simulink model "Displays_ARES_Sim"  (R2019b)
settings: Solver=FixedStepAuto  StartTime=0  StopTime=500  RelTol=1e-3  EnableMultiTasking=on
values from neighbouring files (symbols this model uses):
  Avail_Mode = 2    [Init_Vars_ARES_Sim.m]    (also in Init_Vars_ARES_Sim_SR.m = 0; Init_Vars_ARES_Sim_SR_Michael.m = 0)
  quad_s = 1    [Init_Vars_ARES_Sim.m]    (also in Init_Vars_ARES_Sim_SR.m; Init_Vars_ARES_Sim_SR_Michael.m)
  xLP0 = x0    (= 12000)    [Init_Vars_ARES_Sim.m]    (also in Init_Vars_ARES_Sim_SR.m; Init_Vars_ARES_Sim_SR_Michael.m)
  yLP0 = y0 + 1350    (= 13350)    [Init_Vars_ARES_Sim.m]    (also in Init_Vars_ARES_Sim_SR.m = 10950; Init_Vars_ARES_Sim_SR_Michael.m = 10950)
undefined symbols (not defined in the file or in its folder): LPs, var
libraries: vrlib x37, simulink x5, visionsources x3, simulink_extras x1, aerolibanimutils x1
(part 2 of 2)

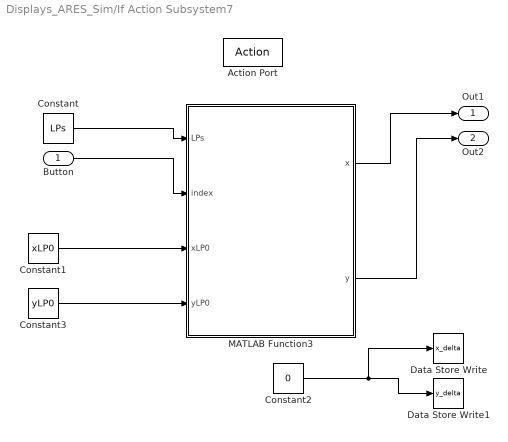
== system Displays_ARES_Sim/If Action Subsystem7 ==
  Button : Inport
  Action Port : ActionPort  ActionPortLabel=if(u1 ~= 0)
  Constant : Constant  Value=LPs
  Constant1 : Constant  Value=xLP0
  Constant2 : Constant  Value=0
  Constant3 : Constant  Value=yLP0
  Data Store Write : DataStoreWrite  DataStoreName=x_delta
  Data Store Write1 : DataStoreWrite  DataStoreName=y_delta
  MATLAB Function3 : MATLAB Function  TreatAsAtomicUnit=on
  Out1 : Outport  InitialOutput=[xLP0]  VectorParamsAs1DForOutWhenUnconnected=off
  Out2 : Outport  Port=2  InitialOutput=[yLP0]  VectorParamsAs1DForOutWhenUnconnected=off
  wires:
  Constant1/1 -> MATLAB Function3/3(xLP0)
  Constant/1 -> MATLAB Function3/1(LPs)
  Constant3/1 -> MATLAB Function3/4(yLP0)
  Button/1 -> MATLAB Function3/2(index)
  MATLAB Function3/1(x) -> Out1/1
  MATLAB Function3/2(y) -> Out2/1
  Constant2/1 -> Data Store Write1/1, Data Store Write/1

== system Displays_ARES_Sim/If Action Subsystem8 ==
  Action Port : ActionPort  ActionPortLabel=if(u1 < 0.0003)

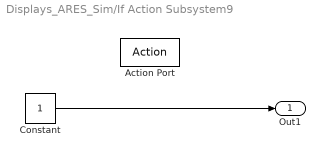
== system Displays_ARES_Sim/If Action Subsystem9 ==
  Action Port : ActionPort  ActionPortLabel=if(u1 ==1 & u2 ==1)
  Constant : Constant
  Out1 : Outport  InitialOutput=[0]  VectorParamsAs1DForOutWhenUnconnected=off
  wires:
  Constant/1 -> Out1/1

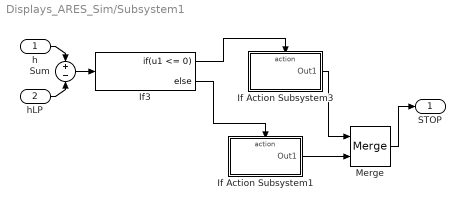
== system Displays_ARES_Sim/Subsystem1 ==
  h : Inport
  hLP : Inport  Port=2
  If Action Subsystem1 : Subsystem  TreatAsAtomicUnit=on
  If Action Subsystem3 : Subsystem  TreatAsAtomicUnit=on
  If3 : If  IfExpression=u1 <= 0  ZeroCross=off
  Merge : Merge
  Sum : Sum  Inputs=+-
  STOP : Outport  VectorParamsAs1DForOutWhenUnconnected=off
  wires:
  If3/1 -> If Action Subsystem3/Action
  Sum/1 -> If3/1
  h/1 -> Sum/1
  hLP/1 -> Sum/2
  If3/2 -> If Action Subsystem1/Action
  If Action Subsystem3/1(Out1) -> Merge/1
  Merge/1 -> STOP/1
  If Action Subsystem1/1(Out1) -> Merge/2

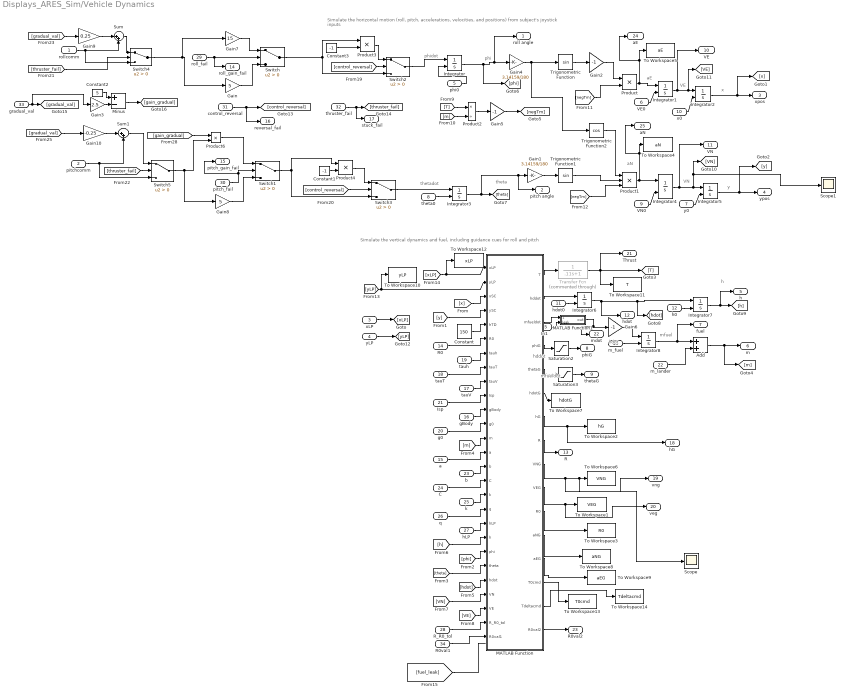
== system Displays_ARES_Sim/Vehicle Dynamics  ==
  note: Simulate the horizontal motion (roll, pitch, accelerations, velocities, and positions) from subject's joystick inputs
  note: Simulate the vertical dynamics and fuel, including guidance cues for roll and pitch
  note: mfuel
  note: mfueldot
  note: h
  note: hdot
  note: hddot
  note: aN
  note: x
  note: VE
  note: aE
  note: phi
  note: phidot
  note: theta
  note: thetadot
  note: y
  note: VN
  rollcomm : Inport
  "pitchcomm " : Inport  Port=2
  xLP : Inport  Port=3
  yLP : Inport  Port=4
  phi0 : Inport  Port=5
  VE0 : Inport  Port=6
  y0 : Inport  Port=7
  "theta0 " : Inport  Port=8
  VN0 : Inport  Port=9
  "x0 " : Inport  Port=10
  hdot0 : Inport  Port=11
  h0 : Inport  Port=12
  m_fuel : Inport  Port=13
  R0 : Inport  Port=14
  a : Inport  Port=15
  gBody : Inport  Port=16
  tauV : Inport  Port=17
  tauT : Inport  Port=18
  tauh : Inport  Port=19
  g0 : Inport  Port=20
  Isp : Inport  Port=21
  m_lander : Inport  Port=22
  "b " : Inport  Port=23
  C : Inport  Port=24
  k : Inport  Port=25
  q : Inport  Port=26
  hLP : Inport  Port=27
  R_R0_tol : Inport  Port=28
  roll_fail : Inport  Port=29
  pitch_fail : Inport  Port=30
  control_reversal : Inport  Port=31
  thruster_fail : Inport  Port=32
  gradual_val : Inport  Port=33
  R0val1 : Inport  Port=34
  In1 : Inport  Port=35
  Add : Sum
  Constant : Constant  Value=150
  Constant1 : Constant  Value=-1
  Constant2 : Constant  Value=5
  Constant3 : Constant  Value=-1
  Gain : Gain  Gain=5
  Gain1 : Gain  Gain=3.14159/180
  Gain10 : Gain  Gain=-0.25
  Gain2 : Gain  Gain=-1
  Gain3 : Gain  Gain=2.5
  Gain4 : Gain  Gain=3.14159/180
  Gain5 : Gain  Gain=-1
  Gain6 : Gain  Gain=-1
  Gain7 : Gain  Gain=15
  Gain8 : Gain  Gain=5
  Gain9 : Gain  Gain=0.25
  Integrator{,1,6..8} (5 alike) : Integrator  InitialConditionSource=external
  Integrator2 : Integrator  InitialConditionSource=external  InitialCondition=1000
  Integrator3 : Integrator  InitialConditionSource=external  InitialCondition=-16
  Integrator4 : Integrator  InitialConditionSource=external  InitialCondition=var]
  Integrator5 : Integrator  InitialConditionSource=external  InitialCondition=1000
  MATLAB Function : MATLAB Function  TreatAsAtomicUnit=on  SystemSampleTime=0.1
  MATLAB Function1 : MATLAB Function  TreatAsAtomicUnit=on
  Minus : Sum  Inputs=+-
  Product{,3..4,6} (4 alike) : Product
  Product1 : Product  Inputs=3
  Product2 : Product  Inputs=*/
  Saturation2 : Saturate  UpperLimit=45  LowerLimit=-45
  Saturation3 : Saturate  UpperLimit=45  LowerLimit=-45
  Scope : Scope
  Scope1 : Scope
  Sum : Sum  Inputs=|++
  Sum1 : Sum  Inputs=|++
  Switch{,1..5} (6 alike) : Switch  Criteria=u2 > Threshold
  To Workspace1 : ToWorkspace  VariableName=VEG  SaveFormat=Timeseries  SampleTime=-1
  To Workspace10 : ToWorkspace  VariableName=yLP  SaveFormat=Timeseries  SampleTime=-1
  To Workspace11 : ToWorkspace  VariableName=T  SaveFormat=Timeseries  SampleTime=-1
  To Workspace12 : ToWorkspace  VariableName=xLP  SaveFormat=Timeseries  SampleTime=-1
  To Workspace13 : ToWorkspace  VariableName=T0cmd  SaveFormat=Timeseries  SampleTime=-1
  To Workspace14 : ToWorkspace  VariableName=Tdeltacmd  SaveFormat=Timeseries  SampleTime=-1
  To Workspace2 : ToWorkspace  VariableName=hG  SaveFormat=Timeseries  SampleTime=-1
  To Workspace3 : ToWorkspace  VariableName=R0  SaveFormat=Timeseries  SampleTime=-1
  To Workspace4 : ToWorkspace  VariableName=aN  SaveFormat=Timeseries  SampleTime=-1
  To Workspace5 : ToWorkspace  VariableName=aE  SaveFormat=Timeseries  SampleTime=-1
  To Workspace6 : ToWorkspace  VariableName=VNG  SaveFormat=Timeseries  SampleTime=-1
  To Workspace7 : ToWorkspace  VariableName=hdotG  SaveFormat=Timeseries  SampleTime=-1
  To Workspace8 : ToWorkspace  VariableName=aNG  SaveFormat=Timeseries  SampleTime=-1
  To Workspace9 : ToWorkspace  VariableName=aEG  SaveFormat=Timeseries  SampleTime=-1
  Transfer Fcn : TransferFcn  Commented=through  Denominator=[.11 1]
  Trigonometric Function : Trigonometry
  Trigonometric Function1 : Trigonometry
  Trigonometric Function2 : Trigonometry  Operator=cos
  roll angle : Outport  VectorParamsAs1DForOutWhenUnconnected=off
  pitch angle : Outport  Port=2  VectorParamsAs1DForOutWhenUnconnected=off
  xpos : Outport  Port=3  VectorParamsAs1DForOutWhenUnconnected=off
  "ypos " : Outport  Port=4  VectorParamsAs1DForOutWhenUnconnected=off
  h : Outport  Port=5  VectorParamsAs1DForOutWhenUnconnected=off
  m : Outport  Port=6  VectorParamsAs1DForOutWhenUnconnected=off
  fuel : Outport  Port=7  VectorParamsAs1DForOutWhenUnconnected=off
  phiG : Outport  Port=8  VectorParamsAs1DForOutWhenUnconnected=off
  thetaG : Outport  Port=9  VectorParamsAs1DForOutWhenUnconnected=off
  VE : Outport  Port=10  VectorParamsAs1DForOutWhenUnconnected=off
  VN : Outport  Port=11  VectorParamsAs1DForOutWhenUnconnected=off
  "hdot " : Outport  Port=12  VectorParamsAs1DForOutWhenUnconnected=off
  R : Outport  Port=13  VectorParamsAs1DForOutWhenUnconnected=off
  roll_gain_fail : Outport  Port=14  VectorParamsAs1DForOutWhenUnconnected=off
  pitch_gain_fail : Outport  Port=15  VectorParamsAs1DForOutWhenUnconnected=off
  reversal_fail : Outport  Port=16  VectorParamsAs1DForOutWhenUnconnected=off
  stuck_fail : Outport  Port=17  VectorParamsAs1DForOutWhenUnconnected=off
  hG : Outport  Port=18  VectorParamsAs1DForOutWhenUnconnected=off
  "vng " : Outport  Port=19  VectorParamsAs1DForOutWhenUnconnected=off
  veg : Outport  Port=20  VectorParamsAs1DForOutWhenUnconnected=off
  Thrust : Outport  Port=21  VectorParamsAs1DForOutWhenUnconnected=off
  mdot : Outport  Port=22  VectorParamsAs1DForOutWhenUnconnected=off
  R0val2 : Outport  Port=23  VectorParamsAs1DForOutWhenUnconnected=off
  aE : Outport  Port=24  VectorParamsAs1DForOutWhenUnconnected=off
  aN : Outport  Port=25  VectorParamsAs1DForOutWhenUnconnected=off
  wires:
  Trigonometric Function/1 -> Gain2/1
  Product/1 -> aE/1, To Workspace5/1, Integrator1/1
  Integrator1/1 -> VE/1, [VE], Integrator2/1
  Integrator2/1 -> xpos/1, [x]
  Gain2/1 -> Product/1
  [negTm] -> Product1/3
  Trigonometric Function1/1 -> Product1/2
  Trigonometric Function2/1 -> Product1/1
  Integrator4/1 -> VN/1, Scope1/1, [VN], Integrator5/1
  Integrator5/1 -> "ypos "/1, [y]
  Product1/1 -> aN/1, To Workspace4/1, Integrator4/1
  MATLAB Function/2(hddot) -> Integrator6/1
  xLP/1 -> [xLP]
  yLP/1 -> [yLP]
  [x] -> MATLAB Function/3(xSC)
  [y] -> MATLAB Function/4(ySC)
  R0/1 -> MATLAB Function/6("R0 ")
  tauh/1 -> MATLAB Function/7(tauh)
  Integrator7/1 -> h/1, [h]
  Add/1 -> m/1, [m]
  Gain6/1 -> Integrator8/1
  Integrator8/1 -> fuel/1, Add/1
  m_lander/1 -> Add/2
  [T] -> Product2/1
  Product2/1 -> Gain5/1
  Gain5/1 -> [negTm]
  [negTm] -> Product/2
  phi0/1 -> Integrator/2
  VE0/1 -> Integrator1/2
  y0/1 -> Integrator5/2
  "theta0 "/1 -> Integrator3/2
  VN0/1 -> Integrator4/2
  "x0 "/1 -> Integrator2/2
  h0/1 -> Integrator7/2
  hdot0/1 -> Integrator6/2
  m_fuel/1 -> Integrator8/2
  tauT/1 -> MATLAB Function/8(tauT)
  Isp/1 -> MATLAB Function/10(Isp)
  gBody/1 -> MATLAB Function/11(gBody)
  g0/1 -> MATLAB Function/12(g0)
  [m] -> MATLAB Function/13(m)
  [h] -> MATLAB Function/20(h)
  [phi] -> MATLAB Function/21(phi)
  [hdot] -> MATLAB Function/23(hdot)
  [theta] -> MATLAB Function/22(theta)
  [VN] -> MATLAB Function/24(VN)
  [VE] -> MATLAB Function/25(VE)
  tauV/1 -> MATLAB Function/9(tauV)
  [m] -> Product2/2
  MATLAB Function/8(R) -> R/1
  Gain1/1 -> Trigonometric Function1/1
  Gain4/1 -> Trigonometric Function2/1, Trigonometric Function/1
  "b "/1 -> MATLAB Function/15(b)
  C/1 -> MATLAB Function/16(C)
  k/1 -> MATLAB Function/17(k)
  Integrator/1 -> [phi], roll angle/1, Gain4/1
  Integrator3/1 -> pitch angle/1, Gain1/1, [theta]
  Constant/1 -> MATLAB Function/5(hTD)
  hLP/1 -> MATLAB Function/19(hLP)
  q/1 -> MATLAB Function/18(q)
  a/1 -> MATLAB Function/14(a)
  MATLAB Function/4(phiG) -> Saturation2/1
  Saturation2/1 -> phiG/1
  MATLAB Function/5(thetaG) -> Saturation3/1
  Saturation3/1 -> thetaG/1
  MATLAB Function/9(VNG) -> Scope/1, "vng "/1, To Workspace6/1
  MATLAB Function/6(hdotG) -> To Workspace7/1
  MATLAB Function/7(hG) -> hG/1, To Workspace2/1
  [xLP] -> MATLAB Function/1(xLP), To Workspace12/1
  [yLP] -> To Workspace10/1, MATLAB Function/2(yLP)
  R_R0_tol/1 -> MATLAB Function/26(R_R0_tol)
  MATLAB Function/11(R0) -> To Workspace3/1
  MATLAB Function/12(aNG) -> To Workspace8/1
  MATLAB Function/13(aEG) -> To Workspace9/1
  MATLAB Function/14(T0cmd) -> To Workspace13/1
  MATLAB Function/15(Tdeltacmd) -> To Workspace14/1
  MATLAB Function/1(T) -> Transfer Fcn/1
  Integrator6/1 -> [hdot], Integrator7/1, "hdot "/1
  Gain/1 -> Switch/3
  Gain8/1 -> Switch1/3
  roll_fail/1 -> roll_gain_fail/1, Switch/2
  pitch_fail/1 -> pitch_gain_fail/1, Switch1/2
  Constant3/1 -> Product3/2
  Switch2/1 -> Integrator/1
  control_reversal/1 -> reversal_fail/1, [control_reversal]
  [control_reversal] -> Switch2/2
  Product3/1 -> Switch2/1
  Switch/1 -> Switch2/3, Product3/1
  Constant1/1 -> Product4/2
  [control_reversal] -> Switch3/2
  Product4/1 -> Switch3/1
  Switch3/1 -> Integrator3/1
  Switch1/1 -> Switch3/3, Product4/1
  Sum/1 -> Switch4/1
  thruster_fail/1 -> [thruster_fail], stuck_fail/1
  rollcomm/1 -> Sum/2, Switch4/3
  [thruster_fail] -> Switch4/2
  [thruster_fail] -> Switch5/2
  "pitchcomm "/1 -> Switch5/3, Sum1/2
  Sum1/1 -> Switch5/1
  Switch4/1 -> Gain7/1, Gain/1
  Gain9/1 -> Sum/1
  [gradual_val] -> Gain9/1
  [gradual_val] -> Gain10/1
  Gain10/1 -> Sum1/1
  Product6/1 -> Switch1/1
  Switch5/1 -> Product6/2, Gain8/1
  gradual_val/1 -> Gain3/1, [gradual_val]
  Constant2/1 -> Minus/1
  Gain3/1 -> Minus/2
  Minus/1 -> [gain_gradual]
  [gain_gradual] -> Product6/1
  MATLAB Function/10(VEG) -> veg/1, To Workspace1/1
  Transfer Fcn/1 -> To Workspace11/1, Thrust/1, [T]
  Gain7/1 -> Switch/1
  R0val1/1 -> MATLAB Function/27(R0val1)
  MATLAB Function/16(R0val2) -> R0val2/1
  [fuel_leak] -> ?
  MATLAB Function/3(mfueldot) -> MATLAB Function1/1(mfueldot)
  MATLAB Function1/1(out) -> mdot/1, Gain6/1
  In1/1 -> MATLAB Function1/2(leak)

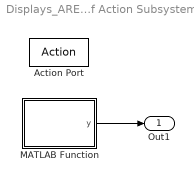
== system Displays_ARES_Sim/If Action Subsystem5/If Action Subsystem1 ==
  Action Port : ActionPort  ActionPortLabel=elseif(u1 == 2)
  MATLAB Function : MATLAB Function  TreatAsAtomicUnit=on
  Out1 : Outport  VectorParamsAs1DForOutWhenUnconnected=off
  wires:
  MATLAB Function/1(y) -> Out1/1

== system Displays_ARES_Sim/If Action Subsystem5/If Action Subsystem2 ==
  Action Port : ActionPort  ActionPortLabel=if(u1 == 1)
  MATLAB Function : MATLAB Function  TreatAsAtomicUnit=on
  Out1 : Outport  VectorParamsAs1DForOutWhenUnconnected=off
  wires:
  MATLAB Function/1(y) -> Out1/1

== system Displays_ARES_Sim/If Action Subsystem5/If Action Subsystem3 ==
  Action Port : ActionPort  ActionPortLabel=elseif( u1 == 3)
  MATLAB Function : MATLAB Function  TreatAsAtomicUnit=on
  Out1 : Outport  VectorParamsAs1DForOutWhenUnconnected=off
  wires:
  MATLAB Function/1(y) -> Out1/1

== system Displays_ARES_Sim/If Action Subsystem5/If Action Subsystem4 ==
  Action Port : ActionPort  ActionPortLabel=elseif( u1 == 4)
  MATLAB Function : MATLAB Function  TreatAsAtomicUnit=on
  Out1 : Outport  VectorParamsAs1DForOutWhenUnconnected=off
  wires:
  MATLAB Function/1(y) -> Out1/1

== system Displays_ARES_Sim/If Action Subsystem5/If Action Subsystem5 ==
  Action Port : ActionPort  ActionPortLabel=elseif(u1==5)
  MATLAB Function : MATLAB Function  TreatAsAtomicUnit=on
  Out1 : Outport  VectorParamsAs1DForOutWhenUnconnected=off
  wires:
  MATLAB Function/1(y) -> Out1/1

== system Displays_ARES_Sim/If Action Subsystem5/If Action Subsystem6 ==
  Action Port : ActionPort  ActionPortLabel=elseif(u1==6)
  MATLAB Function : MATLAB Function  TreatAsAtomicUnit=on
  Out1 : Outport  VectorParamsAs1DForOutWhenUnconnected=off
  wires:
  MATLAB Function/1(y) -> Out1/1

== system Displays_ARES_Sim/Subsystem1/If Action Subsystem1 ==
  Action Port : ActionPort  ActionPortLabel=else
  Constant1 : Constant  Value=0
  Out1 : Outport  VectorParamsAs1DForOutWhenUnconnected=off
  wires:
  Constant1/1 -> Out1/1

== system Displays_ARES_Sim/Subsystem1/If Action Subsystem3 ==
  Action Port : ActionPort  ActionPortLabel=if(u1 <= 0)
  Constant1 : Constant
  Out1 : Outport  InitialOutput=[0]  VectorParamsAs1DForOutWhenUnconnected=off
  wires:
  Constant1/1 -> Out1/1

== matlab function Displays_ARES_Sim/If Action Subsystem/Fuel Gauge ==
  data: fuel input; pts output; m_fuel0 input; fuel_percent output
function [pts,fuel_percent] = fcn( fuel, m_fuel0 )
pts = [0 0 0];
fuelH = fuel/m_fuel0;
fuel_percent = fuelH;
p9 = [ 1 fuelH 1];

pts = [p9];

== matlab function Displays_ARES_Sim/Vehicle Dynamics /MATLAB Function ==
  settings: updateMethod=DISCRETE
  data: xLP input; T output; yLP input; xSC input; ySC input; hTD input; R0 input; tauh input; tauT input; tauV input; Isp input; gBody input; g0 input; m input; a input; b input; C input; k input; q input; hLP input; hddot output; mfueldot output; h input; phi input; theta input; hdot input; VN input; VE input; phiG output; thetaG output; hdotG output; hG output; R output; VNG output; VEG output; R_R0_tol input; R0 output; aNG output; aEG output; T0cmd output; Tdeltacmd output; R0val data_store_memory; R0val1 input; R0val2 output
function [T, hddot, mfueldot, phiG, thetaG, hdotG, hG, R, VNG, VEG,R0,aNG,aEG,T0cmd,Tdeltacmd,R0val2]= fcn(xLP, yLP, xSC, ySC, hTD, R0,tauh, tauT, tauV, Isp, gBody, g0, m, a, b, C, k, q, hLP, h, phi, theta, hdot, VN, VE, R_R0_tol,R0val1)


%% Guidance 
ySC_LP = ySC - yLP; % north distance in s/c to LP
xSC_LP = xSC - xLP; % east distance in s/c to LP
hRel = h - hLP;
psi = 0;

R = sqrt(xSC_LP^2 + ySC_LP^2);

R0 = R0val1;

% Our added logic to deal with cases where you are farther away from LP
% than when you started the landing
if (R/R0val1) > (exp(1)^2 - R_R0_tol)
    % Change R0 to your actual range because VN blows up  if R/R0 is
    % greater than e^2. This will create a "new" simulation (new initial
    % range that you are evaluating from). Essentially  restarting the
    % simulation where the previous state left of
    % Set R0 global to the current range value (redefine R0) (new R0 for
    % the remaining time steps)
    R0val2 = R;
    % Changes R0 for the current time step
    R0 = R;
%     Rchecker = 1;
else
    R0val2 = R0val1;
end

% changed from -xSC and -ySC
angleLP = 180/pi*atan2(-xSC_LP,-ySC_LP);
Rdot = -VN*cosd(angleLP) - VE*sind(angleLP);

% Hdot Guidance
if hRel >= 150
    hG = C + (((hTD-C)^log(sqrt(R/R0)))/k)^(1/(log(sqrt(R/R0))-1));     % ft, Equation 10
    if hG > 1000
        hG = 1000;
    end
    hdotG = (a*hG + b) + (hG - hRel)/tauh;                               % ft/s, Equation 11
else
    hG = hRel;     % ft, not a real thing, just a place holder for once we get below 150 ft since hG is no longer defined
    hdotG = -3;                                                       % ft, if below 150 ft, just descend at -3 ft/s
end

% Add in a limit that if we are too far away (>Rlim) but too low (<150ft),
% go into hover (this is our own personal addition, not from Bilimoria)
Rlim = 100; %50     % ft, the limit for how small the range has to be for us to continue to descend if we are below 150 ft
if hRel < hTD && R > Rlim
    hdotG = 0;  % go into a hover (i.e. hdotG=0)
end

% Limit hdotG to between 0 and -30 f/s
if hdotG > 0
    hdotG = 0;
elseif hdotG < -16
    hdotG = -16;
end

% Define a deadband that will be added in on the Tdetlacmd when assum
hdot_deadband = 0.1;                % ft/s
% The commanded vertical velocity will always be the guidance vertical velocity

hdotcmd = hdotG;        % assuming this to be the case, need to verify

%% hdotG failure...
% if no_fail 
% hdotcmd = hdotG;        % assuming this to be the case, need to verify
% else
%     hdotcmd = 1.3*hdot
% end
%% 

% thrust command
T0cmd = m*gBody/(cosd(theta)*cosd(phi));       % ft-lbs (like N), Equation 1, primary thrust command to counteract weight of the vehicle
% change in thrust command
Tdeltacmd = m/(cosd(theta)*cosd(phi)) * (hdotcmd-hdot)/tauT;    % ft-lbs (like N), Equation 2, secondary thrust command to adjust descent rate
% Add a deadband in on the Tdetlacmd
if abs(hdotcmd-hdot) < hdot_deadband
    Tdeltacmd = 0;
end
T = T0cmd + Tdeltacmd; % ft-lbs (like N), total thrust command
% Constrain thrust between 10% and 60% of max operational thrust (10,000 lbf)
if T > 6000
    T = 6000;
end
if T < 1000
    T = 1000;
end
hddot = T/m * cosd(phi)*cosd(theta) - gBody;    % ft/s^2, vertical acceleration
% Change in vehicle mass
mfueldot = T/(Isp*g0);      % slugs/s, fuel consumption rate, assumes ideal rocket equation
% mdot = -mfueldot;           % slug/s
% if fuel_leak==1
%     mfueldot=1.5*mfueldot;
% end 

% Velocity guidance (North and East)
VNG = ySC_LP*q*(1-log(sqrt(R/R0)));     % ft/s, Equation 13a
VEG = xSC_LP*q*(1-log(sqrt(R/R0)));     % ft/s, Equation 13b

% acceleration Guidance (North and East)
% Set x acceleration equal to zero if x = 0
if ySC_LP == 0
    aNG = 0;
else
    aNG = (VN*VNG/ySC_LP + q*(-1)*ySC_LP*Rdot/(2*R)) + (VNG - VN)/tauV;  % ft/s^2, Equation 15a
end
% Set y acceleration equal to zero if y = 0
if xSC_LP == 0
    aEG = 0;
else
    aEG = (VE*VEG/xSC_LP + q*(-1)*xSC_LP*Rdot/(2*R)) + (VEG - VE)/tauV;  % ft/s^2, Equation 15b
end

temp = -m/T * (aNG*sind(psi) - aEG*cosd(psi));
if temp > 1
    temp = 1;
elseif temp < -1
    temp = -1;
end

% % roll Guidance
phiG = asind(temp);   % deg, (positive is nose up), Equation 17a
% % Limit phiG by +/- 45 deg
if phiG > 45
    phiG = 45;
elseif phiG < -45
    phiG = -45;
end

% Limit phiG by +/- 30 deg to try and make trials longer
% if phiG > 30
%     phiG = 30;
% elseif phiG < -30
%     phiG = -30;
% end


temp2 = -m/(T*cosd(phiG)) * (aNG*cosd(psi) + aEG*sind(psi));
if temp2 > 1
    temp2 = 1;
elseif temp2 < -1
    temp2 = -1;
end

% pitch Guidance
thetaG = asind(temp2);   % deg, (positive is nose up), Equation 17b
% % Limit thetaG by +/- 45 deg
if thetaG > 45
    thetaG = 45;
elseif thetaG < -45
    thetaG = -45;

% Limit thetaG by +/- 30 deg
% if thetaG > 30
%     thetaG = 30;
% elseif thetaG < -30
%     thetaG = -30;
    
end

== matlab function Displays_ARES_Sim/Background Translation ==
  data: pitch input; pts output; roll input
%%%%%%%%%%%%%%%%%%%%%%%%%%%%%%%%%%%%%
% This function is used to define the translation of the guidance cues
% Elliott Davis 
% Edited: 4/30/18
% Joshua Seedorf
% Edited: 1/21/20
% Modified transformation to display roll correctly
%%%%%%%%%%%%%%%%%%%%%%%%%%%%%%%%%%%%%
function pts   = fcn( pitch, roll )

% Roll and Pitch
% x = xy(1);
% y = xy(2);

%% Roll Correction
% X-component
x = (0.1045)*pitch*sind(roll);
% Y-component
y = (0.1045)*pitch*cosd(roll);

% Output for VR sink (y,z)
% pts = [0 (-pitch-25) -.5];
pts = [x -y-25 -0.5];

== matlab function Displays_ARES_Sim/Rotations ==
  data: xy input; pts output
%%%%%%%%%%%%%%%%%%%%%%%%%%%%%%%%%%%%%
% This function is used to define the rotation of pitch bars
% Elliott Davis 
% Edited: 4/30/18
%%%%%%%%%%%%%%%%%%%%%%%%%%%%%%%%%%%%%
function pts   = fcn( xy )

% Roll and Pitch
x = xy(1);
y = xy(2);

% Output for VR sink (z,angle)
pts = [ 1 x/5.75];

== matlab function Displays_ARES_Sim/Guidance Cross ==
  data: thetaG input; pts output; phiG input; theta input; phi input
%%%%%%%%%%%%%%%%%%%%%%%%%%%%%%%%%%%%%
% This function is used to define the translation of the guidance cues
% Elliott Davis 
% Edited: 4/30/18
%%%%%%%%%%%%%%%%%%%%%%%%%%%%%%%%%%%%%
function pts = fcn( thetaG, phiG, theta, phi )

% Input pitch/roll and respective guidance
x = phiG;
y = thetaG;
out1 = x-phi;
out2 = y-theta;

% Define limits on the outputs
if out1 >= 4.5
    out1 = 4.5;
elseif out1 <= -4.5 
    out1 = -4.5;
end 

if out2 >= 4.5
    out2 = 4.5;
elseif out2 <= -4.5 
    out2 = -4.5;
end 

% Output for VR sink (x,y,z)
pts = [out1 out2 .001];

== matlab function Displays_ARES_Sim/Roll Triangle ==
  data: xy input; pts output; gradual input; fail input
%%%%%%%%%%%%%%%%%%%%%%%%%%%%%%%%%%%%%
% This function is used to define the subjects roll in the top roll bar 
% Elliott Davis 
% Edited: 4/30/18
%%%%%%%%%%%%%%%%%%%%%%%%%%%%%%%%%%%%%

%%%%% Original
% function pts   = fcn( xy )
% % imageSize = 1000;
% % s = imageSize / 15;
% x = xy(1);
% y = xy(2);
% 
% % Output for VR sink (x,y)
% pts = [x/10 .31];

function pts   = fcn( xy,gradual ,fail )
% imageSize = 1000;
% s = imageSize / 15;
if fail==true 
    x = xy(1)*(1-gradual);
else
    x = xy(1);
end 
    
    
y = xy(2);

% Output for VR sink (x,y)
pts = [x/10 .31];

== matlab function Displays_ARES_Sim/Alt Triangle Pts ==
  data: h input; pts output
%%%%%%%%%%%%%%%%%%%%%%%%%%%%%%%%%%%%%
% This function is used to define the current altitude on the side bar
% Elliott Davis 
% Edited: 4/30/18
%%%%%%%%%%%%%%%%%%%%%%%%%%%%%%%%%%%%%
function pts = fcn(h)

% Define the height of the altitude bar in VR sink terms. 
if h == 125
   Alt = 0;
else 
   Alt = (h-125)/125; 
end

% Output for VR sink (x,y)
pts = [5.5 Alt];

== matlab function Displays_ARES_Sim/MATLAB Function10 ==
  data: time input
function fcn(time)
coder.extrinsic('CallTactile')
if time==1 
    
    CallTactile(.1,5,.5);
end

== matlab function Displays_ARES_Sim/Pitch Translation Bars ==
  data: pitch input; pts output; roll input
%%%%%%%%%%%%%%%%%%%%%%%%%%%%%%%%%%%%%
% This function is used to define the translation of pitch bars
% Elliott Davis 
% Edited: 4/30/18
% Joshua Seedorf
% Edited: 1/23/20
% Modified to properly display roll
%%%%%%%%%%%%%%%%%%%%%%%%%%%%%%%%%%%%%
function pts = fcn(pitch, roll)

% Roll and Pitch
% x = xy(1);
% y = xy(2);

x = (0.1002)*pitch*sind(roll);
y = (0.1)*pitch*cosd(roll);

% Output for VR sink (y)
% pts = [-y];
pts = [x -y];

== matlab function Displays_ARES_Sim/MATLAB Function15 ==
  data: time input; y output; auditory input
function y  = fcn(time,auditory)
y=0;
coder.extrinsic('now')
if time ==0 || auditory==1
    y=now;
end

== matlab function Displays_ARES_Sim/Pitch TranslationText ==
  data: pitch input; pts output; roll input
%%%%%%%%%%%%%%%%%%%%%%%%%%%%%%%%%%%%%
% This function is used to define the translation of pitch text
% Elliott Davis 
% Edited: 4/30/18
%%%%%%%%%%%%%%%%%%%%%%%%%%%%%%%%%%%%%
function pts = fcn(pitch, roll)

% Roll and Pitch
% x = xy(1);
% y = .1*xy(2);

x = (0.0101)*pitch*sind(roll);
y = (0.01)*pitch*cosd(roll);

% Output for VR sink (y)
% pts = [ -y ];
pts = [x -y];

== matlab function Displays_ARES_Sim/Abort_Value_Func1 ==
  data: buttons input; Abort output
function Abort = fcn(buttons)    

        Abort = buttons(2);
end

== matlab function Displays_ARES_Sim/Vehicle Dynamics /MATLAB Function1 ==
  data: mfueldot input; out output; leak input
function out = fcn(mfueldot,leak)
out=mfueldot;
if leak==1
    out=1.1*mfueldot;
end 
end

== matlab function Displays_ARES_Sim/MATLAB Function ==
  data: time input; y output; tactor input; Amp input; dur input
function y = myBlock(time,tactor,Amp,dur)
% Defines usePhyton as an extrisical function and uses it to run
% CallTactile and create a buzz. 

% Daniel Gutierrez-Mendoza
out=0;
coder.extrinsic('usePython');
out=usePython(time,tactor,Amp,dur);
y = out;
end

== matlab function Displays_ARES_Sim/MATLAB Function16 ==
  data: start_time input; time input; leak input; out output
function out =fcn(start_time,time,leak)
coder.extrinsic('Alarm_Bad')
out=0;
if time==0
    Alarm_Bad(start_time);
elseif leak==0 && time>start_time
    out=1;
end

== matlab function Displays_ARES_Sim/Define Buttons LPs1 ==
  data: buttons input; button output; button_IPC output; total output; Mode output; auditory output
function [button, button_IPC, total, Mode,auditory]  = fcn(buttons)
% This function reads in the array 'buttons' from the stick and decides if
% a button was pressed and which one it was.
% 
% 
% Test = buttons(1); % Trigger
% Test = buttons(2); % Safety
% Test = buttons(3); % Button A
% Test = buttons(4); % Button B
% Test = buttons(5); % Button C
% Test = buttons(6); % Bottom Trigger
% Test = buttons(7); % Button D
% Test = buttons(8); % Button E
% Test = buttons(9); % T1
% Test = buttons(10); % T2
% Test = buttons(11); % T3
% Test = buttons(12); % T4
% Test = buttons(13); % T5
% Test = buttons(14); % T6
% Test = buttons(15); % Trigger Second Detent
% Test = buttons(16); % Stick upper trim UP
% Test = buttons(17); % Stick upper trim Right
% Test = buttons(18); % Stick upper trim Down
% Test = buttons(19); % Stick upper trim Left
% Test = buttons(20); % Throttle index switch UP
% Test = buttons(21); % Throttle index switch Right
% Test = buttons(22); % Throttle index switch Down
% Test = buttons(23); % Throttle index switch Left
% Test = buttons(24); % Throttle Small gray button (does not reset to 0)
% Test = buttons(25); % Mode Select,  Mode 2 = 1
% Test = buttons(26); % Mode Select, Mode 3 = 1
% Test = buttons(27); % Throttle FUNCTION button
% Test = buttons(28); % Throttle START/STOP button
% Test = buttons(29); % Throttle RESET button
% Test = buttons(30); % Throttle 'i' button
% Test = buttons(31); % Throttle Small gray button (does reset to 0)
% Test = buttons(32); %Throttle wheel press
% Test = buttons(33); %Throttle wheel forward
% Test = buttons(34); %Throttle wheel backward

% 'total' sums the binary values coming from each of the six LP buttons.
% This value is used in deciding if a button was pressed.
total = (buttons(9) + buttons(10) + buttons(11) +buttons(12)+buttons(13)...
    +buttons(14)+buttons(3));
%total_IPC = (buttons(16) + buttons(17) + buttons(18) +buttons(19));

% Control Mode Selection
if buttons (25) == 1
    Mode = 1; % RCAH +IPC
    IPC_active = 1;
elseif buttons(26) == 1
    Mode = 2; % IPC
    IPC_active =1;
else
    Mode = 0; % RCAH
    IPC_active = 0;
end

% Small Landing Point correction 

if buttons(16) == 1
    button_IPC = 1;
elseif buttons(18) == 1
    button_IPC = 2;
elseif buttons(17) == 1
    button_IPC = 3;
elseif buttons(19) == 1
    button_IPC = 4;
else
    button_IPC = 0;
end

% Landing Point selection 
if buttons(9)==1
    button = 1;
elseif buttons(10)==1
    button = 2;
elseif buttons(11)==1
    button = 3;
elseif buttons(12)==1
    button = 4;
elseif buttons(13)==1
    button = 5;
elseif buttons(14)==1
    button = 6;

else
    button=0;
    
end

% Audiory Stuff 
auditory=0;
if buttons(30)==1
    auditory=1;
end 

   
    
   
    
   
    
    
   
end

== matlab function Displays_ARES_Sim/AUTO Mode Select1 ==
  data: Mode input; xy output; R input
% Carlos Pinedo
% 4/21/2020
% Control Mode Color Selection IPC Logic
function xy   = Mode_Sel_AUTO(Mode, R)
Rauto = 350;
if Mode == 2
    xy = [ 0.9 0.1 1.0];
elseif Mode == 1 && R < Rauto
    xy = [1 0.7 0.2];
else
     xy = [1 1 0];
end

== matlab function Displays_ARES_Sim/MATLAB Function7 ==
  data: u input; ON output; first_buzz_start_time input; Mag output; dur output; sec_time input
function [ON,Mag,dur] = TactileONFF(u,first_buzz_start_time,sec_time)
% This makes decides if the tactile buzzes or not at an instant and
% determines the magnitude of the buzz. Also defines the duration of the
% buzz. 

% Daniel Gutierrez-Mendoza 

coder.extrinsic('ExtrinsicStepsTactile');
dur=.5;
ON=0;
Mag=0;
[ON,Mag,dur]=ExtrinsicStepsTactile(u,dur,first_buzz_start_time,sec_time);
end

== matlab function Displays_ARES_Sim/MATLAB Function17 ==
  data: u input
function  fcn(u)
coder.extrinsic('Stopit')
Stopit(u);

== matlab function Displays_ARES_Sim/MATLAB Function18 ==
  data: time input; out output; start_time input; auditory_press input
function out = fcn(time,start_time,auditory_press)
out=0;
if time>start_time
    out=auditory_press;
else 
    out=0;
end

== matlab function Displays_ARES_Sim/Secondary Workload ==
  data: buttons input; Detected output; fail_detect input; fail_button output
function [Detected,fail_button] = fcn(buttons,fail_detect)

%Test = buttons(1); % Trigger
%Test = buttons(2); % Safety
%Test = buttons(3); % Button A
%Test = buttons(4); % Button B
%Test = buttons(5); % Button C
%Test = buttons(6); % Bottom Trigger
%Test = buttons(7); % Button D
%Test = buttons(8); % Button E
fail_button = buttons(7);

if fail_detect==1
    Detected = buttons(7);
else 
    Detected=false;
end

== matlab function Displays_ARES_Sim/Designated Landing ==
  data: heightLP input; pts output
%%%%%%%%%%%%%%%%%%%%%%%%%%%%%%%%%%%%%
% This function is used to define the landing site height in VR sink
% Elliott Davis 
% Edited: 4/30/18
%%%%%%%%%%%%%%%%%%%%%%%%%%%%%%%%%%%%%
function pts = fcn(heightLP)

% Define the height of the landing site in VR sink terms
if heightLP == 125
    heightLPDisp = 0;
else 
    heightLPDisp = (heightLP-125)/125; 
end

% Output for VR sink (x,y,z)
pts = [5.5 heightLPDisp .01];

== matlab function Displays_ARES_Sim/MATLAB Function5 ==
  data: t output
%  This Function Returns the Current Computer Time
% Created by: Nicholas Miller
%
% This function creates a timeseries within simulink, where the
% left column is simulation time and the right column is the actual time in
% serial date number.
   
function t = sysClock

eml.extrinsic('now');
t=0;
t = now;

end

== matlab function Displays_ARES_Sim/B&E function1 ==
  settings: updateMethod=DISCRETE
  data: t input; status output; fail_time output
%%%%%%%%%%%%%%%%%%%%%%%%%%%%%%%%%%%%%%%%%%%%%%%%%%%%%%%%%%%%%%%%%%%%%%%%
% This function compares the simulation time to pre-generated pseudorandom
% times for the secondary workload assessment (B&E test).
% Joshua Seedorf
% Created: 1/17/20
%%%%%%%%%%%%%%%%%%%%%%%%%%%%%%%%%%%%%%%%%%%%%%%%%%%%%%%%%%%%%%%%%%%%%%%%
function [status,fail_time] = secondary_workload_function(t)
% Vector of test times was generated using Generate_B_E_test_times.m
times = [14,26,39,57,73,93,106,126,143,155,171,189,205,223,240];

% Max duration for each test 
dt = 10; %seconds

% ACII(66) => "B"
% status = uint8(66); %"B"
%status = uint8(70); %"F"
status = uint8(8);
% Compare time to the vector of test times
for x = 1:length(times)
    if t >= times(x) && t <= times(x)+dt
        % ACII(69) => "E"
        %status = uint8(69);
        status = uint8(3);
        %fail_time = times(x);
        break
    end
end
fail_time = times(x);

== matlab function Displays_ARES_Sim/Designated hTD ==
  data: height_hTD input; pts output
%%%%%%%%%%%%%%%%%%%%%%%%%%%%%%%%%%%%%
% This function is used to define the terminal descent point
% Elliott Davis 
% Edited: 4/30/18
%%%%%%%%%%%%%%%%%%%%%%%%%%%%%%%%%%%%%
function pts = fcn(height_hTD)

% The terminal descent point in VR sink terms
if height_hTD == 125
    height_hTD_Disp = 0;
else 
    height_hTD_Disp = (height_hTD-125)/125; 
end

% Output for VR sink (x,y,z)
pts = [5.5 height_hTD_Disp .01];

== matlab function Displays_ARES_Sim/Guidance Triangle ==
  data: pts output; phiG input; phi input
%%%%%%%%%%%%%%%%%%%%%%%%%%%%%%%%%%%%%
% This function is used to define the subjects guidance roll in the top 
% roll bar 
% Elliott Davis 
% Edited: 4/30/18
%%%%%%%%%%%%%%%%%%%%%%%%%%%%%%%%%%%%%
function pts = fcn(  phiG, phi )
% imageSize = 1000;
% s = imageSize / 15;

% Define ranges of guidance roll triangle in top roll bar
x = phiG;

if x >= 4.5
    x = 4.6;
elseif x <= -4.5 
    x = -4.6;
end 

% Output for VR sink (x,y,z)
pts = [x/10 .355 9.1];

== matlab function Displays_ARES_Sim/MATLAB Function1 ==
  data: Time input
function fcn(Time)


if Time == 0
    pause(.3)
    
%     coder.extrinsic('udp_communication_start');
%     udp_communication_start();    
%     
end

== matlab function Displays_ARES_Sim/If Action Subsystem6/MATLAB Function3 ==
  data: x output; xLP input; y output; yLP input; x_delta input; y_delta input; button_IPC input; interval input; x_delta output; y_delta output; Mode input; R input
function [x,y,x_delta,y_delta] = fcn(xLP,yLP,x_delta,y_delta,button_IPC,interval,Mode,R)
% Has a LP redesignation occured if yes, interval reset to zero
% if total == 1
%     interval = 0;
% end
if Mode > 0
%     if sqrt(x_delta^2 + y_delta^2) > 300
%         x_delta = x_delta + 0;
%         y_delta = y_delta + 0;
    if button_IPC == 1  % Y-Pos
        x_delta = x_delta + 0;
        y_delta = y_delta + interval;
    elseif button_IPC == 2 % X-Pos
        %         x_delta = x_delta + interval;
        %         y_delta = y_delta + 0;
        x_delta = x_delta + 0;
        y_delta = y_delta - interval;
    elseif button_IPC == 3 % Y-Neg
        %         x_delta = x_delta + 0;
        %         y_delta = y_delta - interval;
        x_delta = x_delta + interval;
        y_delta = y_delta + 0;
    elseif button_IPC == 4 % X-Neg
        x_delta = x_delta - interval;
        y_delta = y_delta + 0;
        %     else
        %         x_delta = x_delta + 0;
        %         y_delta = y_delta + 0;
    end
    
    
  
%     
% else
%     x = xLP;
%     y = yLP;
end
 if x_delta > 300
     x_delta = 300;
 end
 if x_delta < -300
     x_delta = -300;
 end
 if y_delta > 300
     y_delta = 300;
 end
 if y_delta < -300
     y_delta = -300;
 end
   x = xLP + x_delta;
    y = yLP+ y_delta;
end

== matlab function Displays_ARES_Sim/If Action Subsystem5/If Action Subsystem2/MATLAB Function ==
  data: y output
  function y = fcn()

y = [1;0;0;0;0;0];

== matlab function Displays_ARES_Sim/If Action Subsystem5/If Action Subsystem1/MATLAB Function ==
  data: y output
  function y = fcn()

y = [0;1;0;0;0;0];

== matlab function Displays_ARES_Sim/MATLAB Function3 ==
  data: mdot input; fuel input
function time_to_empty(mdot,fuel)

te = fuel/mdot;

% Get vrworld associated with the VR Sink found there
wh=vrworld(get_param('PFD_HSD_ARES_Realtime_Latest_Version/VR Sink1', 'VRWorld1.wrl'));
% Handle to the Text node we want to control
nh=vrnode(wh,'Time_Display');
% Set the new value of the 'string' field of the Text node)
% the string can be a vector of strings
setfield(nh, 'string', strcat(num2str(te)),'s');

== matlab function Displays_ARES_Sim/If Action Subsystem5/If Action Subsystem3/MATLAB Function ==
  data: y output
  function y = fcn()

y = [0;0;1;0;0;0];

== matlab function Displays_ARES_Sim/If Action Subsystem5/If Action Subsystem4/MATLAB Function ==
  data: y output
  function y = fcn()

y = [0;0;0;1;0;0];

== matlab function Displays_ARES_Sim/If Action Subsystem5/If Action Subsystem5/MATLAB Function ==
  data: y output
  function y = fcn()

y = [0;0;0;0;1;0];

== matlab function Displays_ARES_Sim/MATLAB Function4 ==
  data: VE input; heading output; VN input
%%%%%%%%%%%%%%%%%%%%%%%%%%%%%%%%%%%%%%%%%%%%%%%%%%%%%%%%%%%%%%%%%%%%%%%%
% Joshua Seedorf
% Created: 1/21/20
%%%%%%%%%%%%%%%%%%%%%%%%%%%%%%%%%%%%%%%%%%%%%%%%%%%%%%%%%%%%%%%%%%%%%%%%
function heading = determine_heading(VE,VN)
heading = atand(abs(VE/VN));

if VE < 0
    heading = -heading;
end

if VN < 0
    heading = 180 - heading;
end

== matlab function Displays_ARES_Sim/If Action Subsystem5/If Action Subsystem6/MATLAB Function ==
  data: y output
  function y = fcn()

y = [0;0;0;0;0;1];

== matlab function Displays_ARES_Sim/Groundspeed ==
  data: v input; y output
%Joshua Seedorf
%2/17/2020
%Converts groundspeed for use in VRWorld
function y = speed2pix(v)

ypos = v*(2.94/150) - 2.94;

y = [-4.7 ypos 0.15];

== matlab function Displays_ARES_Sim/Vertical Rate ==
  data: hdot input; y output
%Joshua Seedorf
%2/18/2020
%Converts hdot for use in VRWorld
function y = vert2pix(hdot)

y = hdot*(2.94/21) - 0.2;

== matlab function Displays_ARES_Sim/If Action Subsystem7/MATLAB Function3 ==
  data: x output; LPs input; y output; index input; xLP0 input; yLP0 input
function [x,y] = fcn(LPs,index,xLP0,yLP0)



    
    if index == 0
        x = xLP0;
        y = yLP0;
    else
        x = LPs(1,index);
        y = LPs(2,index);
    end


end

== matlab function Displays_ARES_Sim/HSI_Acc1 ==
  data: VEG input; xy output; VNG input
% Joshua Seedorf
% 4/12/2020
% Acceleration conversion for HSI
function xy   = hsi_VG(VEG,VNG)
xy = [VEG VNG]/10;

if norm(xy) >= 3
    xy = 3*(xy./norm(xy));
end

== matlab function Displays_ARES_Sim/HSI_Ball ==
  data: VN input; xy output; VE input
% Joshua Seedorf
% 2/18/2020
% Velocity conversion for HSI
function xy = hsi_ball(VN,VE)
xy = [VE VN]/100;

if norm(xy) >= 3
    xy = 3*(xy./norm(xy));
end

== matlab function Displays_ARES_Sim/MATLAB Function6 ==
  data: speed input; mode output; R input; pitch_com input; roll_com input; buttons input; Avail_Mode input
function mode = ipctrans(speed,R,pitch_com,roll_com,buttons,Avail_Mode)
% Joshua Seedorf
%   5/11/2020
% Function for automated IPC transition

% Modes
rcah = 0;
mipc = 1;
aipc = 2;

% Mode initialize
mode = 0;

% Factors
Vmax = 40; %[ft/s]d
Ripc = 500; %[ft]
Rauto = 350; %[ft]
defmax = 0.325; %[joystick deflection]

%% Mode Transitions
% Total combined deflection
def = sqrt(pitch_com^2+roll_com^2);
% Sum of landing point buttons to detect any selections
total = (buttons(9) + buttons(10) + buttons(11) +buttons(12)+buttons(13)...
    +buttons(14)+buttons(3));
if Avail_Mode == 0 %rcah only
    mode = rcah;
elseif Avail_Mode == 1 %rcah + IPA
    if speed < Vmax && total == 0 && R < Ripc
        mode = mipc;
    else
        mode = rcah;
    end
    
elseif Avail_Mode == 2 % rcah + IPC
    if  speed < Vmax && def < defmax && total == 0
        if  R < Rauto
            mode = aipc;
        elseif R < Ripc
            mode = mipc;
%         elseif R < Rauto && def > defmax
%             mode = mipc;
        else
            mode = rcah;
        end
%     elseif total == 0
%         if speed < Vmax && R < Ripc && def < defmax
%             mode = aipc;
%         elseif R < Ripc
%             mode = mipc;
%         else
%             mode = rcah;
%         end
    elseif speed < Vmax && R < Ripc && total == 0
        mode = mipc;
    else
        mode = rcah;
    end
end

== matlab function Displays_ARES_Sim/MATLAB Function2 ==
  data: u input; y output; s input
function y = fcn(u,s)
% This is the function that was used to derive the equation of the failure
% function:
% 
% v3 = spline([9 11], [0.25 2.25 4 1.5]);
% plot(linspace(9, 11), ppval(v3, linspace(9,11)), 'm--')
% 
% u = current time in seconds
% s = failure time in seconds
% 
% The failure function:

if u < s
    y = 0;
    
elseif u < s+9
    y = 0.25*(u-s);
    
elseif u < s+11
    y = 0.3125*(u-(s+9))^2 + 0.25*(u-(9+s)) + 2.25;
    
elseif u < s+15
    y = (1.5)*(u-s) - 12.5;
    
else
    y = 10;
    
end

y = y/10;

end

== matlab function Displays_ARES_Sim/MATLAB Function9 ==
  data: h input; z_abort output; hLP input; abort input; fuel input; z_land output; z_fuel output
function [z_abort,z_land,z_fuel] = hsi_stop_img(h,hLP,abort,fuel)

if h <= hLP+0.25
    z_land = 0.2;
else
    z_land = -1;
end

if abort
    z_abort = 0.2;
else
    z_abort = -1;
end

if fuel <= 0.05
    z_fuel = 0.19;
else
    z_fuel = -1;
end

== matlab function Displays_ARES_Sim/MATLAB Function11 ==
  data: theta input; y output
function y = fcn(theta)
theta = abs(theta);
if theta > 6
    y = 2;
elseif theta > 3
    y = 1;
else 
    y = 0;
end

== matlab function Displays_ARES_Sim/MATLAB Function8 ==
  data: h input; Abort_true output boolean
function Abort_true = fcn(h)
% Set Abort Window
if h <=200 && h >=50
    Abort = 1;
else
    Abort = 0;
end
Abort_true = logical(Abort);

== matlab function Displays_ARES_Sim/MATLAB Function12 ==
  data: theta input; y output
function y = fcn(theta)
theta = abs(theta);
if theta > 6
    y = 2;
elseif theta > 3
    y = 1;
else 
    y = 0;
end

== matlab function Displays_ARES_Sim/MATLAB Function13 ==
  data: theta input; y output
function y = fcn(theta)
theta = abs(theta);
if theta > 4
    y = 2;
elseif theta > 2
    y = 1;
else 
    y = 0;
end

== matlab function Displays_ARES_Sim/MATLAB Function14 ==
  data: XLP input; og_lp output; YLP input; avail_mode input
% Function for displaying the original LP on HSI
% Joshua Seedorf
% 8/18/2020
function og_lp = hsi_ald(XLP,YLP,avail_mode)

if avail_mode > 0
    og_lp = [XLP/100,YLP/100,-0.011];
else
    og_lp = [XLP/100,YLP/100,-10];
end

== matlab function Displays_ARES_Sim/time_to_empty ==
  data: tte output; m input; m_Lander input
%%%%%%%%%%%%%%%%%%%%%%%%%%%%%%%%%%%%%
% Estimates the time to empty
% Joshua Seedorf
% Edited: 4/12/20
%%%%%%%%%%%%%%%%%%%%%%%%%%%%%%%%%%%%%
function tte   = fcn( m,m_Lander )
% Cubic fit to a time remaining vs fuel curve
fit = [-0.022397, 3.858436];
m_f = m-m_Lander;
tte = round(fit(1).*m_f.^2 + fit(2).*m_f.^1);

== matlab function Displays_ARES_Sim/HSI_LP ==
  data: range output; theta output; xyLP output; dLPX input; dLPY input; xyHSI output
% Joshua Seedorf
% 2/18/2020
% LP conversion for HSI
function [range,theta,xyLP,xyHSI]  = hsi_LP(dLPX,dLPY)
range = round(norm([dLPX dLPY]));
xyHSI = [0,0];
xyHSI = [dLPX dLPY]/100;
theta = atan(dLPX/dLPY);

if norm(xyHSI) >= 3
    xyLP = 3*(xyHSI./norm(xyHSI));
else
    xyLP = xyHSI;
end

if dLPY < 0
    theta = theta + pi;
end

== matlab function Displays_ARES_Sim/HSI_VG ==
  data: VEG input; xy output; VNG input
% Joshua Seedorf
% 2/19/2020
% Guidance velocity conversion for HSI
function xy   = hsi_VG(VEG,VNG)
xy = [VEG VNG]/100;

if norm(xy) >= 3
    xy = 3*(xy./norm(xy));
end

== matlab function Displays_ARES_Sim/HSI_Vec ==
  data: theta output; scale output; VN input; xy output; VE input
% Joshua Seedorf
% 2/18/2020
% Velocity conversion for HSI
function [theta,scale,xy] = hsi_vec(VN,VE)
xy = [VE VN]/200;
scale = norm(xy)/10;
theta = atan(VN/VE) + pi/2;

if norm(xy) >= 1.5
    xy = 1.5*(xy./norm(xy));
    scale = 1.5/10;
end

== matlab function Displays_ARES_Sim/AUTO Mode Select3 ==
  data: Mode input; xy output; R input
% Carlos Pinedo
% 4/21/2020
% Control Mode Color Selection IPC Logic
function xy   = Mode_Sel_IPC_AUTO(Mode,R)
Rauto = 350;
if Mode == 2
    xy = [ 0 1 0];
elseif Mode == 1 && R < Rauto
    xy = [1 0.7 0.2];
else
     xy = [0.8 0.8 0.8];
end

== matlab function Displays_ARES_Sim/IPC Mode Select2 ==
  data: Mode input; xy output
% Carlos Pinedo
% 4/21/2020
% Control Mode Color Selection IPC Logic
function xy   = Mode_Sel_IPC(Mode)

if Mode == 1
    
    xy = [ 0 1 0];
else
    xy = [0.8 0.8 0.8];
end

== matlab function Displays_ARES_Sim/RCAH Mode Select1 ==
  data: Mode input; xy output
% Carlos Pinedo
% 4/21/2020
% Control Mode Color Selection RCAH Logic
function xy   = Mode_Sel_RCAH(Mode)

if Mode == 2
    xy = [0.8 0.8 0.8];
else
    xy = [ 0 1 0];
end
